simulink model "LDOPowerModel"  (R2018a)
settings: Solver=ode23t  StartTime=0.0  StopTime=20  MaxStep=1e-4  RelTol=1e-3
libraries: fl_lib x12, nesl_utility x9
settings Model: Creator=kamranhasan  LastModifiedBy=xulingx1
settings DebuggingCC: MaxConsecutiveZCsMsg=none
settings CodeAppCC: StateflowObjectComments=on
settings SimscapeCC: SimscapeNormalizeSystem=off

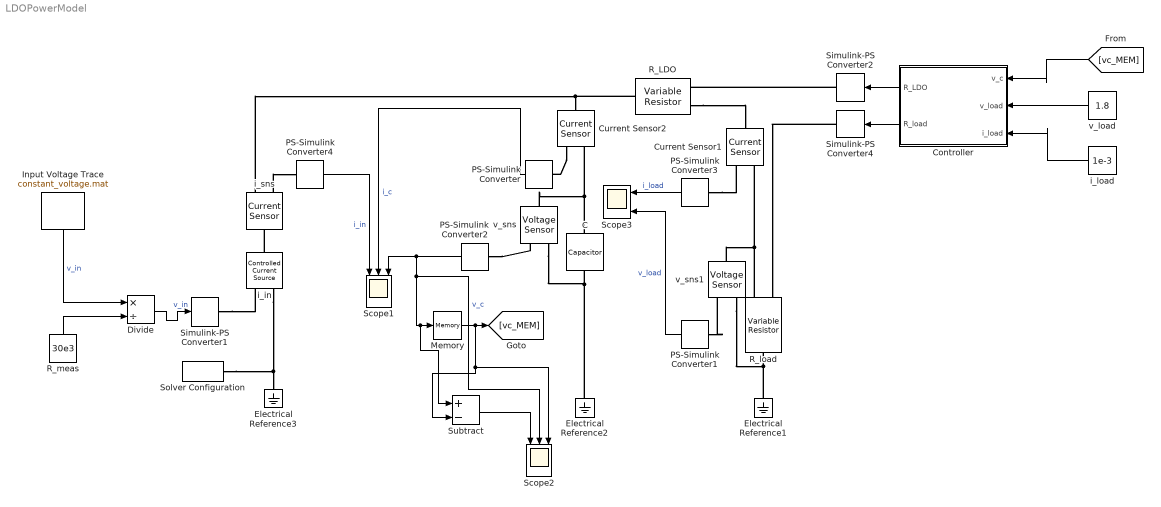
== system LDOPowerModel ==
  C : fl_lib/Electrical/Electrical Elements/Capacitor  c=10e-6 F  r=0 Ohm  g=0 1/Ohm  i_specify=off  i_priority=None  i=0 A  i_nominal_specify=off  i_nominal_unit=A  i_nominal_value=1  v_specify=off  v_priority=None  v=0 V  v_nominal_specify=off  v_nominal_unit=V  v_nominal_value=1  vc_specify=off  vc_priority=High  vc=0 V  vc_nominal_specify=off  vc_nominal_unit=V  vc_nominal_value=1
  Controller : MATLAB Function  Priority=1  TreatAsAtomicUnit=on
  Current Sensor1 : fl_lib/Electrical/Electrical Sensors/Current Sensor
      settings: SourceProductName=Foundation Library
  Current Sensor2 : fl_lib/Electrical/Electrical Sensors/Current Sensor
      settings: SourceProductName=Foundation Library
  Divide : Product  Inputs=*/
  Electrical Reference1 : fl_lib/Electrical/Electrical Elements/Electrical Reference
  Electrical Reference2 : fl_lib/Electrical/Electrical Elements/Electrical Reference
  Electrical Reference3 : fl_lib/Electrical/Electrical Elements/Electrical Reference
  Input Voltage Trace : FromFile  FileName=constant_voltage.mat  SampleTime=0.001  ExtrapolationBeforeFirstDataPoint=Hold first value  InterpolationWithinTimeRange=Zero order hold  ExtrapolationAfterLastDataPoint=Hold last value
  Memory : Memory
  PS-Simulink Converter : nesl_utility/PS-Simulink Converter  PhysicalDomain=network_engine_domain  SubClassName=ps_output  LeftPortType=input  RightPortType=output  PseudoPeriodic=off  Frequencies=[]  Unit=A  AffineConversion=off
  PS-Simulink Converter1 : nesl_utility/PS-Simulink Converter  PhysicalDomain=network_engine_domain  SubClassName=ps_output  LeftPortType=input  RightPortType=output  PseudoPeriodic=off  Frequencies=[]  Unit=V  AffineConversion=off
  PS-Simulink Converter2 : nesl_utility/PS-Simulink Converter  PhysicalDomain=network_engine_domain  SubClassName=ps_output  LeftPortType=input  RightPortType=output  PseudoPeriodic=off  Frequencies=[]  Unit=V  AffineConversion=off
  PS-Simulink Converter3 : nesl_utility/PS-Simulink Converter  PhysicalDomain=network_engine_domain  SubClassName=ps_output  LeftPortType=input  RightPortType=output  PseudoPeriodic=off  Frequencies=[]  Unit=1  AffineConversion=off
  PS-Simulink Converter4 : nesl_utility/PS-Simulink Converter  PhysicalDomain=network_engine_domain  SubClassName=ps_output  LeftPortType=input  RightPortType=output  PseudoPeriodic=off  Frequencies=[]  Unit=A  AffineConversion=off
  R_LDO : fl_lib/Electrical/Electrical Elements/Variable Resistor  Rmin=1e-9 Ohm  i_specify=off  i_priority=None  i=0 A  i_nominal_specify=off  i_nominal_unit=A  i_nominal_value=1  v_specify=off  v_priority=None  v=0 V  v_nominal_specify=off  v_nominal_unit=V  v_nominal_value=1
  R_load : fl_lib/Electrical/Electrical Elements/Variable Resistor  Rmin=1e-9 Ohm  i_specify=off  i_priority=None  i=0 A  i_nominal_specify=off  i_nominal_unit=A  i_nominal_value=1  v_specify=off  v_priority=None  v=0 V  v_nominal_specify=off  v_nominal_unit=V  v_nominal_value=1
  R_meas : Constant  Value=30e3
  Scope1 : Scope  NumInputPorts=3
  Scope2 : Scope  NumInputPorts=3
  Scope3 : Scope  NumInputPorts=2
  Simulink-PS Converter1 : nesl_utility/Simulink-PS Converter  PhysicalDomain=network_engine_domain  SubClassName=ps_input  LeftPortType=input  RightPortType=output  PseudoPeriodic=off  Frequencies=[]  NoiseDistribution=none  NoiseParameters=[]  Unit=1  AffineConversion=off  FilteringAndDerivatives=provide  SimscapeFilterOrder=1  InputFilterTimeConstant=0.001  UdotUserProvided=0
  Simulink-PS Converter2 : nesl_utility/Simulink-PS Converter  PhysicalDomain=network_engine_domain  SubClassName=ps_input  LeftPortType=input  RightPortType=output  PseudoPeriodic=off  Frequencies=[]  NoiseDistribution=none  NoiseParameters=[]  Unit=1  AffineConversion=off  FilteringAndDerivatives=provide  SimscapeFilterOrder=1  InputFilterTimeConstant=0.001  UdotUserProvided=0
  Simulink-PS Converter4 : nesl_utility/Simulink-PS Converter  PhysicalDomain=network_engine_domain  SubClassName=ps_input  LeftPortType=input  RightPortType=output  PseudoPeriodic=off  Frequencies=[]  NoiseDistribution=none  NoiseParameters=[]  Unit=1  AffineConversion=off  FilteringAndDerivatives=provide  SimscapeFilterOrder=1  InputFilterTimeConstant=0.001  UdotUserProvided=0
  Solver Configuration : nesl_utility/Solver Configuration  PhysicalDomain=network_engine_domain  SubClassName=solver  LeftPortType=input  RightPortType=generic  Tones=[]  Harmonics=[]  SimulateNoise=on  Profile=off  UseLocalSampling=off  EnableSwitchedLinearOptims=on  FrequencyDomain=off  UseCCode=off  RelTol=0.001  AbsTol=1e-06  MinStep=1e-09  ToWorkspace=off  RevertToSquareIcSolve=off  NumHomotopyIterations=100  PhasorMode=off  PhasorModeNumHarmonics=1  DoDC=off  ResidualTolerance=1e-9  UseLocalSolver=on  LocalSolverChoice=NE_BACKWARD_EULER_ADVANCER  LocalSolverSampleTime=.00001  DoFixedCost=on  MaxNonlinIter=3  MaxModeIter=2  LinearAlgebra=Sparse  EquationFormulation=NE_TIME_EF  DelaysMemoryBudget=1024  AutomaticFiltering=on  FilteringTimeConstant=0.001
  Subtract : Sum  Inputs=+-
  i_in : fl_lib/Electrical/Electrical Sources/Controlled Current Source
  i_load : Constant  Value=1e-3
  i_sns : fl_lib/Electrical/Electrical Sensors/Current Sensor
      settings: SourceProductName=Foundation Library
  v_load : Constant  Value=1.8
  v_sns : fl_lib/Electrical/Electrical Sensors/Voltage Sensor
  v_sns1 : fl_lib/Electrical/Electrical Sensors/Voltage Sensor
  wires:
  Input Voltage Trace/1 -> Divide/1  "v_in"
  R_meas/1 -> Divide/2
  PS-Simulink Converter/1 -> Scope1/2  "i_c"
  PS-Simulink Converter2/1 -> Scope1/3, Scope2/2, Subtract/1, Memory/1  "v_c"
  PS-Simulink Converter3/1 -> Scope3/1  "i_load"
  PS-Simulink Converter4/1 -> Scope1/1  "i_in"
  Memory/1 -> Subtract/2, Scope2/3, [vc_MEM]
  Divide/1 -> Simulink-PS Converter1/1  "v_in"
  Controller/1(R_LDO) -> Simulink-PS Converter2/1
  Controller/2(R_load) -> Simulink-PS Converter4/1
  v_load/1 -> Controller/2(v_load)
  i_load/1 -> Controller/3(i_load)
  [vc_MEM] -> Controller/1(v_c)
  PS-Simulink Converter1/1 -> Scope3/2  "v_load"
  Subtract/1 -> Scope2/1
  connections:
  R_load/LConn2 -- Current Sensor1/RConn2 -- v_sns1/LConn1
  Electrical Reference1/LConn1 -- v_sns1/RConn2 -- R_load/RConn1
  Electrical Reference2/LConn1 -- v_sns/RConn2 -- C/RConn1
  R_LDO/RConn1 -- i_sns/RConn2 -- Current Sensor2/LConn1
  i_in/RConn2 -- Solver Configuration/RConn1 -- Electrical Reference3/LConn1
  C/LConn1 -- Current Sensor2/RConn2 -- v_sns/LConn1
  Current Sensor2/RConn1 -- PS-Simulink Converter/LConn1
  PS-Simulink Converter2/LConn1 -- v_sns/RConn1
  PS-Simulink Converter3/LConn1 -- Current Sensor1/RConn1
  i_in/LConn1 -- i_sns/LConn1
  i_sns/RConn1 -- PS-Simulink Converter4/LConn1
  Simulink-PS Converter1/RConn1 -- i_in/RConn1
  R_LDO/LConn2 -- Current Sensor1/LConn1
  Simulink-PS Converter2/RConn1 -- R_LDO/LConn1
  Simulink-PS Converter4/RConn1 -- R_load/LConn1
  PS-Simulink Converter1/LConn1 -- v_sns1/RConn1

== matlab function LDOPowerModel/Controller ==
  data: v_c input; R_LDO output; v_load input; i_load input; R_load output
function [R_LDO, R_load] = fcn(v_c, v_load, i_load)
persistent charge_cap
if isempty(charge_cap)
    charge_cap = 1;
end

if (v_c <= 1.80)
   charge_cap = 1; 
elseif (v_c > 4.5)
    charge_cap = 0;
end

if(charge_cap == 1)
    R_LDO  = 1e15;  % simulate infinite resistance (open circuit)
    R_load = 1e-9; % connect load to ground through tiny R to ensure zero current
else %set R_LDO such that v_load is maintained
    R_load = (1.8/1.3e-3);
    R_LDO = (R_load*((v_c) - v_load))/v_load;
end
